simulink model "Just_The_Electrical_model"  (R2016a)
settings: Solver=VariableStepAuto  StartTime=0.0  StopTime=10.0  RelTol=1e-3
values from neighbouring files (symbols this model uses):
  BT = {}    [Electrical_model_settings.m]
  btc = {}    [Electrical_model_settings.m]
  col = {}    [Electrical_model_settings.m]
  elc = {}    [Electrical_model_settings.m]
  ess = {}    [Electrical_model_settings.m]
  fcc = {}    [Electrical_model_settings.m]
  flex = {}    [Electrical_model_settings.m]
  systemBase = {}    [Electrical_model_settings.m]
  wf = {}    [Electrical_model_settings.m]
  wt1 = {}    [Electrical_model_settings.m]
  wt2 = wt1    [Electrical_model_settings.m]
  wt3 = wt1    [Electrical_model_settings.m]
undefined symbols (not defined in the file or in its folder): avr, D1, Delta, DiscIntNeverNeededParam, f2ctrl, governor, interface, Lf1, sm, Ts, Ts_phy, Ts_sim, u0
libraries: powerlib x69, pwrsysBasic x68, simulink_extras x37, pwrsysVICtrl x22, powerlib_meascontrol x19, simulink x8, pwrsysVSrc x5, pwrsysTransf x5, pwrsys-matlab x1
(part 2 of 4)

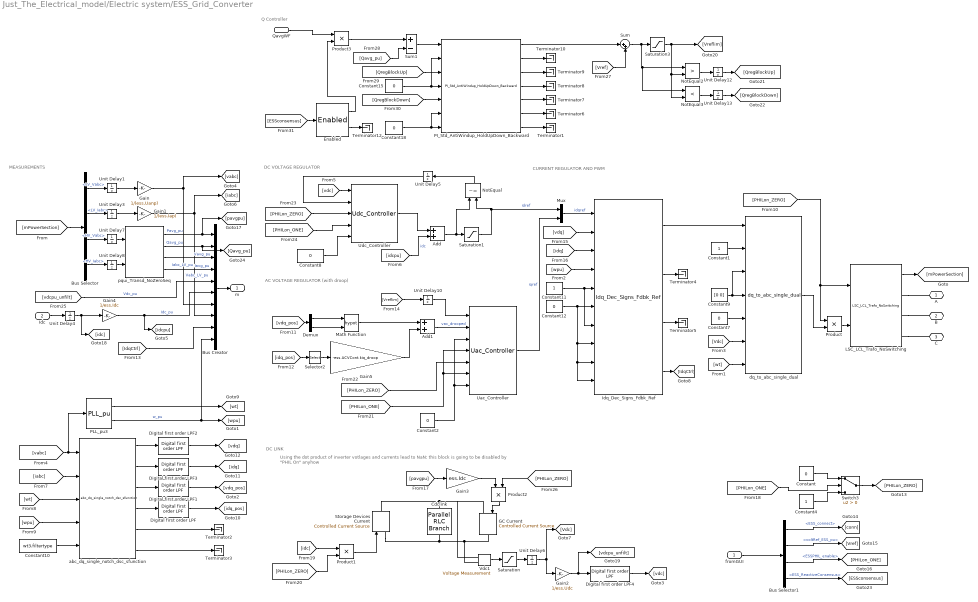
== system Just_The_Electrical_model/Electric system/ESS_Grid_Converter ==
  note: DC LINK
  note: Using the dot product of inverter votlages and currents lead to NaN: this block is going to be disabled by "PHIL On" anyhow
  note: MEASUREMENTS
  note: AC VOLTAGE REGULATOR (with droop)
  note: DC VOLTAGE REGULATOR
  note: CURRENT REGULATOR AND PWM
  note: Q Controller
  fromGUI : Inport
  Idc : Inport  Port=2
  QavgWF : Inport  Port=3
  Add : Sum
  Add1 : Sum
  Bus Creator : BusCreator  Inputs=10
  Bus Selector : BusSelector  OutputSignals=LV_Vabc,LV_Iabc,HV_Vabc,HV_Iabc
  Bus Selector1 : BusSelector  OutputSignals=ESS_connect,voltRef_ESS_pu,ESSPHIL_enable,ESS_ReactiveConsensus
  Cdclink : powerlib/Elements/Parallel RLC Branch  LConnTagsString=a  RConnTagsString=__new0  BranchType=RC  Resistance=1e6  Inductance=0  SetiL0=off  InitialCurrent=0  Capacitance=ess.Cdc  Setx0=on  InitialVoltage=ess.Udc  Measurements=None
  Constant{,2,15,18} (4 alike) : Constant  Value=0
  Constant1 : Constant  SampleTime=ess.Ts_control
  Constant10 : Constant  Value=wt3.filtertype  SampleTime=wt3.Ts_control
  Constant11 : Constant  SampleTime=ess.Ts_control
  Constant12 : Constant  Value=0  SampleTime=ess.Ts_control
  Constant4 : Constant
  Constant7 : Constant  Value=0  SampleTime=ess.Ts_control
  Constant8 : Constant  Value=0  SampleTime=ess.Ts_control
  Constant9 : Constant  Value=[0 0]  SampleTime=ess.Ts_control
  Demux : Demux  Outputs=2
  Digital first order LPF{,1..4} (5 alike) : pwrsysBasic/Digital first order LPF  Ts=ess.Ts_control  fcutout=ess.CurrCont.f_LPF_noise
  Enabled : pwrsysBasic/Enabled
  GC Current : powerlib/Electrical Sources/Controlled Current Source  Initialize=on  Source_Type=DC  Amplitude=0  Phase=0  Frequency=0  Measurements=None
  Gain : Gain  Gain=1/(ess.Uanp)
  Gain1 : Gain  Gain=1/(ess.Iap)
  Gain2 : Gain  Gain=1/ess.Udc
  Gain3 : Gain  Gain=ess.Idc
  Gain4 : Gain  Gain=1/ess.Idc
  Gain5 : Gain  Gain=-ess.ACVCont.kiq_droop
  Idq_Dec_Signs_Fdbk_Ref : pwrsysVICtrl/Idq_Dec_Signs_Fdbk_Ref  Ts=ess.Ts_control  fn=systemBase.fn  Kp=ess.CurrContSingle.kp  Ti=ess.CurrContSingle.Ti  L=ess.CurrCont.x  PI_max=ess.CurrCont.PImax  PI_min=ess.CurrCont.PImin  TrafoPhaseComp=0
  LSC_LCL_Trafo_NoSwitching : pwrsysVSrc/LSC_LCL_Trafo_NoSwitching  Sn=ess.Sn  fn=systemBase.fn  Uhv_ab=systemBase.Vn  Uab=ess.Un  lf2=ess.LCL.l2  rf2=ess.LCL.r2  Lf1=ess.LCL.L1  Rf1=ess.LCL.R1  Cf=ess.LCL.Cf  Rc=ess.LCL.Rf
  Math Function : Math  Operator=hypot  SaturateOnIntegerOverflow=on
  Mux : Mux  Inputs=2
  NotEqual : RelationalOperator  Operator=~=  OutDataTypeStr=boolean
  NotEqual2 : RelationalOperator  Operator=>  OutDataTypeStr=boolean
  NotEqual3 : RelationalOperator  Operator=<  OutDataTypeStr=boolean
  PI_Std_AntiWindup_HoldUpDown_Backward : pwrsysBasic/PI_Std_AntiWindup_HoldUpDown_Backward  Ts=ess.Ts_control  Kg=ess.Qctrl.Kg  Kp=ess.Qctrl.Kp  Ti=ess.Qctrl.Ti  outMax=ess.Qctrl.deltaUmaxPos  outMin=ess.Qctrl.deltaUmaxNeg
  PLL_pu3 : pwrsysBasic/PLL_pu  fn=systemBase.fn  Ts=ess.Ts_control  Kp_pll=90  Ki_pll=1200  Kd_pll=0  PLL_ini=60
  Product{,1..3} (4 alike) : Product
  Saturation : Saturate  UpperLimit=5*ess.Uanp  LowerLimit=0.25*ess.Uanp
  Saturation1 : Saturate  UpperLimit=ess.DCVCont.PImax  LowerLimit=ess.DCVCont.PImin
  Saturation3 : Saturate  UpperLimit=ess.Qctrl.Umax  LowerLimit=ess.Qctrl.Umin
  Selector2 : Selector  IndexMode=Zero-based  InputPortWidth=2  IndexOptions=Index vector (dialog)  Indices=1  OutputSizes=1
  Storage Devices Current : powerlib/Electrical Sources/Controlled Current Source  Initialize=on  Source_Type=DC  Amplitude=0  Phase=0  Frequency=0  Measurements=None
  Sum : Sum  Inputs=|++
  Sum1 : Sum  Inputs=+-
  Switch3 : Switch  Criteria=u2 > Threshold
  Terminator{1..10,12} (11 alike) : Terminator
  Uac_Controller : pwrsysVICtrl/Uac_Controller  Ts=ess.Ts_control  Kg=ess.ACVCont.kg  Kp=ess.ACVCont.kp  Ti=ess.ACVCont.Ti  PI_max=ess.ACVCont.PImax  PI_min=ess.ACVCont.PImin
  Udc_Controller : pwrsysVICtrl/Udc_Controller  Ts=ess.Ts_control  Kp=ess.DCVContSingle.kp  Ti=ess.DCVContSingle.Ti  PI_max=ess.DCVCont.PImax  PI_min=ess.DCVCont.PImin
  Unit Delay{1,3,7..8} (4 alike) : UnitDelay  InitialCondition=[0 0 0]  SampleTime=ess.Ts_control
  Unit Delay10 : UnitDelay  InitialCondition=1  SampleTime=ess.Ts_control
  Unit Delay{4..5,12..13} (4 alike) : UnitDelay  SampleTime=ess.Ts_control
  Unit Delay6 : UnitDelay  InitialCondition=1  SampleTime=ess.Ts_control
  Vdc1 : powerlib/Measurements/Voltage Measurement  PhasorSimulation=off  OutputType=Complex  PSBequivalent=0
  abc_dq_single_notch_dsc_sfunction : pwrsysTransf/abc_dq_single_notch_dsc_sfunction  Ts=ess.Ts_control  fn=2*systemBase.fn  zeta=ess.CurrCont.zeta
  dq_to_abc_single_dual : pwrsysVICtrl/dq_to_abc_single_dual  Ts=ess.Ts_control  Uabp=ess.Uabp
  pqui_Transd_NoZeroSeq : pwrsysBasic/pqui_Transd_NoZeroSeq  Sn=ess.Sn  Uanp=systemBase.Vn*(2/3)^0.5  Iap=ess.Iap*(ess.Un/systemBase.Vn)
  A : PMIOPort  Port=1  Side=Right
  B : PMIOPort  Port=2  Side=Right
  C : PMIOPort  Port=3  Side=Right
  m : Outport
  wires:
  Bus Selector/1 -> Unit Delay1/1  "<LV_Vabc>"
  [idq_pos] -> Selector2/1
  Gain1/1 -> Bus Creator/8, [iabc]  "Iabc_LV_pu"
  Bus Selector/2 -> Unit Delay3/1  "<LV_Iabc>"
  Gain5/1 -> Add1/2
  Math Function/1 -> Add1/1
  [PHILon_ONE] -> Uac_Controller/6, Uac_Controller/4
  Add1/1 -> Uac_Controller/2  "vac_drooped"
  [Vreflim] -> Unit Delay10/1
  [mPowerSection] -> Bus Selector/1
  Gain/1 -> Bus Creator/7, [vabc]  "Vabc_LV_pu"
  [PHILon_ZERO] -> Uac_Controller/5
  Constant8/1 -> Udc_Controller/5
  NotEqual/1 -> Unit Delay5/1
  [vdc] -> Udc_Controller/1
  Unit Delay5/1 -> Udc_Controller/2
  Saturation1/1 -> NotEqual/2, Mux/1  "idref"
  [idcpu] -> Add/2  "idc"
  Udc_Controller/1 -> Add/1
  Add/1 -> NotEqual/1, Saturation1/1
  [PHILon_ZERO] -> Udc_Controller/3
  [idq] -> Idq_Dec_Signs_Fdbk_Ref/3
  [Vdc] -> dq_to_abc_single_dual/6
  [wpu] -> Idq_Dec_Signs_Fdbk_Ref/4
  dq_to_abc_single_dual/1 -> Product/2
  Mux/1 -> Idq_Dec_Signs_Fdbk_Ref/1  "idqref"
  [wt] -> dq_to_abc_single_dual/7
  Constant10/1 -> abc_dq_single_notch_dsc_sfunction/5
  Bus Selector/3 -> Unit Delay7/1  "<HV_Vabc>"
  Bus Selector/4 -> Unit Delay8/1  "<HV_Iabc>"
  pqui_Transd_NoZeroSeq/1 -> [pavgpu], Bus Creator/1  "Pavg_pu"
  pqui_Transd_NoZeroSeq/2 -> [Qavg_pu], Bus Creator/2  "Qavg_pu"
  pqui_Transd_NoZeroSeq/3 -> Bus Creator/3  "Vavg_pu"
  pqui_Transd_NoZeroSeq/4 -> Bus Creator/4  "Iavg_pu"
  Bus Creator/1 -> m/1
  [vdcpu_unfilt] -> Bus Creator/5  "Vdc_pu"
  Gain4/1 -> [idcpu], Bus Creator/6  "Idc_pu"
  PLL_pu3/2 -> Bus Creator/10, [wpu]  "w_pu"
  PLL_pu3/1 -> [wt]
  Uac_Controller/1 -> Mux/2  "iqref"
  LSC_LCL_Trafo_NoSwitching/1 -> [mPowerSection]
  Unit Delay1/1 -> Gain/1
  Unit Delay3/1 -> Gain1/1
  Unit Delay8/1 -> pqui_Transd_NoZeroSeq/2
  Unit Delay7/1 -> pqui_Transd_NoZeroSeq/1
  Unit Delay10/1 -> Uac_Controller/1
  abc_dq_single_notch_dsc_sfunction/6 -> Terminator3/1
  abc_dq_single_notch_dsc_sfunction/5 -> Terminator2/1
  Selector2/1 -> Gain5/1
  Idq_Dec_Signs_Fdbk_Ref/2 -> Terminator4/1
  [vdq] -> Idq_Dec_Signs_Fdbk_Ref/2
  Constant1/1 -> dq_to_abc_single_dual/2
  Constant7/1 -> dq_to_abc_single_dual/5
  Constant9/1 -> dq_to_abc_single_dual/4, dq_to_abc_single_dual/3
  Constant11/1 -> Idq_Dec_Signs_Fdbk_Ref/7, Idq_Dec_Signs_Fdbk_Ref/5
  Constant12/1 -> Idq_Dec_Signs_Fdbk_Ref/8, Idq_Dec_Signs_Fdbk_Ref/9, Idq_Dec_Signs_Fdbk_Ref/10, Idq_Dec_Signs_Fdbk_Ref/6
  Idq_Dec_Signs_Fdbk_Ref/3 -> Terminator5/1
  Idq_Dec_Signs_Fdbk_Ref/4 -> [IdqCtrl]
  [IdqCtrl] -> Bus Creator/9
  Idq_Dec_Signs_Fdbk_Ref/1 -> dq_to_abc_single_dual/1
  [wt] -> abc_dq_single_notch_dsc_sfunction/3
  [wpu] -> abc_dq_single_notch_dsc_sfunction/4
  abc_dq_single_notch_dsc_sfunction/1 -> Digital first order LPF2/1
  [vabc] -> abc_dq_single_notch_dsc_sfunction/1, PLL_pu3/1
  [iabc] -> abc_dq_single_notch_dsc_sfunction/2
  abc_dq_single_notch_dsc_sfunction/3 -> Digital first order LPF1/1
  abc_dq_single_notch_dsc_sfunction/4 -> Digital first order LPF/1
  abc_dq_single_notch_dsc_sfunction/2 -> Digital first order LPF3/1
  Digital first order LPF/1 -> [idq_pos]
  Digital first order LPF1/1 -> [vdq_pos]
  [vdq_pos] -> Demux/1
  Demux/1 -> Math Function/1
  Demux/2 -> Math Function/2
  Digital first order LPF2/1 -> [vdq]
  Digital first order LPF3/1 -> [idq]
  fromGUI/1 -> Bus Selector1/1
  Bus Selector1/1 -> [conn]  "<ESS_connect>"
  Bus Selector1/2 -> [Vref]  "<voltRef_ESS_pu>"
  Idc/1 -> Unit Delay4/1
  Bus Selector1/3 -> [PHILon_ONE]  "<ESSPHIL_enable>"
  Unit Delay4/1 -> [idc], Gain4/1
  Constant/1 -> Switch3/1
  [PHILon_ONE] -> Switch3/2
  Constant4/1 -> Switch3/3
  Switch3/1 -> [PHILon_ZERO]
  [PHILon_ZERO] -> LSC_LCL_Trafo_NoSwitching/1, Product/1
  Product/1 -> LSC_LCL_Trafo_NoSwitching/2
  Gain3/1 -> Product2/1
  [pavgpu] -> Gain3/1
  [idc] -> Product1/1
  Product1/1 -> Storage Devices Current/1
  [PHILon_ZERO] -> Product1/2
  Constant2/1 -> Uac_Controller/3, Uac_Controller/7
  [PHILon_ONE] -> Udc_Controller/4
  Vdc1/1 -> Saturation/1
  Saturation/1 -> Unit Delay6/1
  Unit Delay6/1 -> [Vdc], Gain2/1
  Gain2/1 -> [vdcpu_unfilt], Digital first order LPF4/1
  Digital first order LPF4/1 -> [vdc]
  Product2/1 -> GC Current/1
  [PHILon_ZERO] -> Product2/2
  [Vref] -> Sum/2
  Sum/1 -> NotEqual3/1, NotEqual2/1, Saturation3/1
  Saturation3/1 -> NotEqual3/2, NotEqual2/2, [Vreflim]
  [Qavg_pu] -> Sum1/2
  [ESSconsensus] -> Enabled/1
  [QregBlockUp] -> PI_Std_AntiWindup_HoldUpDown_Backward/3
  Constant15/1 -> PI_Std_AntiWindup_HoldUpDown_Backward/2, PI_Std_AntiWindup_HoldUpDown_Backward/4
  [QregBlockDown] -> PI_Std_AntiWindup_HoldUpDown_Backward/5
  Constant18/1 -> PI_Std_AntiWindup_HoldUpDown_Backward/6, PI_Std_AntiWindup_HoldUpDown_Backward/7
  PI_Std_AntiWindup_HoldUpDown_Backward/7 -> Terminator1/1
  PI_Std_AntiWindup_HoldUpDown_Backward/6 -> Terminator6/1
  PI_Std_AntiWindup_HoldUpDown_Backward/5 -> Terminator7/1
  PI_Std_AntiWindup_HoldUpDown_Backward/4 -> Terminator8/1
  PI_Std_AntiWindup_HoldUpDown_Backward/3 -> Terminator9/1
  PI_Std_AntiWindup_HoldUpDown_Backward/2 -> Terminator10/1
  NotEqual2/1 -> Unit Delay12/1
  Unit Delay12/1 -> [QregBlockUp]
  NotEqual3/1 -> Unit Delay13/1
  Unit Delay13/1 -> [QregBlockDown]
  PI_Std_AntiWindup_HoldUpDown_Backward/1 -> Sum/1
  Bus Selector1/4 -> [ESSconsensus]  "<ESS_ReactiveConsensus>"
  Sum1/1 -> PI_Std_AntiWindup_HoldUpDown_Backward/1
  Enabled/2 -> Terminator12/1
  Product3/1 -> Sum1/1
  QavgWF/1 -> Product3/1
  Enabled/1 -> Product3/2
  connections:
  LSC_LCL_Trafo_NoSwitching/RConn3 -- C/RConn1
  LSC_LCL_Trafo_NoSwitching/RConn1 -- A/RConn1
  LSC_LCL_Trafo_NoSwitching/RConn2 -- B/RConn1
  Storage Devices Current/RConn1 -- Vdc1/LConn1 -- GC Current/LConn1 -- Cdclink/LConn1
  GC Current/RConn1 -- Vdc1/LConn2 -- Storage Devices Current/LConn1 -- Cdclink/RConn1

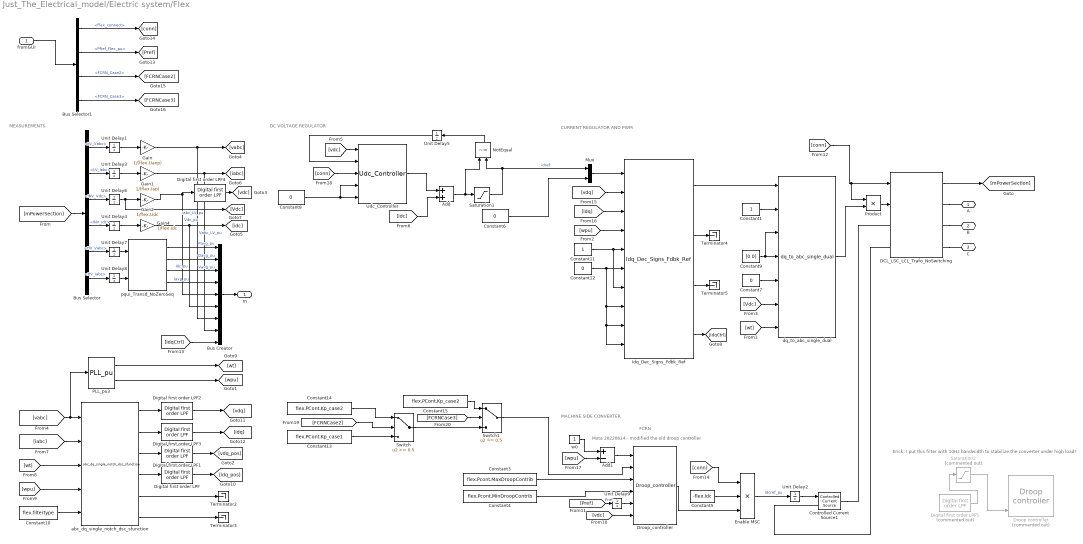
== system Just_The_Electrical_model/Electric system/Flex ==
  note: FCRN
  note: Mota 20220614 - modified the old droop controller
  note: Erick: I put this filter with 10Hz bandwidth to stabilize the converter under high load!
  note: MEASUREMENTS
  note: MACHINE SIDE CONVERTER
  note: DC VOLTAGE REGULATOR
  note: CURRENT REGULATOR AND PWM
  fromGUI : Inport
  Add : Sum
  Add1 : Sum  Inputs=+-
  Bus Creator : BusCreator  Inputs=9
  Bus Selector : BusSelector  OutputSignals=LV_Vabc,LV_Iabc,INV_Vdc,INV_Idc,HV_Vabc,HV_Iabc
  Bus Selector1 : BusSelector  OutputSignals=Flex_connect,PRef_Flex_pu,FCRN_Case2,FCRN_Case3
  Constant1 : Constant  SampleTime=flex.Ts_control
  Constant10 : Constant  Value=flex.filtertype  SampleTime=flex.Ts_control
  Constant11 : Constant  SampleTime=flex.Ts_control
  Constant{6..8,12} (4 alike) : Constant  Value=0  SampleTime=flex.Ts_control
  Constant13 : Constant  Value=flex.PCont.Kp_case1  SampleTime=-1
  Constant14 : Constant  Value=flex.PCont.Kp_case2  SampleTime=-1
  Constant15 : Constant  Value=flex.PCont.Kp_case2  SampleTime=-1
  Constant3 : Constant  Value=flex.Pcont.MaxDroopContrib  SampleTime=flex.Ts_control
  Constant4 : Constant  Value=flex.Pcont.MinDroopContrib  SampleTime=flex.Ts_control
  Constant5 : Constant  Value=-flex.Idc  SampleTime=flex.Ts_control
  Constant9 : Constant  Value=[0 0]  SampleTime=flex.Ts_control
  Controlled Current Source1 : powerlib/Electrical Sources/Controlled Current Source  Initialize=on  Source_Type=DC  Amplitude=0  Phase=0  Frequency=50  Measurements=None
  DCL_LSC_LCL_Trafo_NoSwitching : pwrsysVSrc/DCL_LSC_LCL_Trafo_NoSwitching  Sn=flex.Sn  fn=systemBase.fn  Uhv_ab=systemBase.Vn  Uab=flex.Un  lf2=flex.LCL.l2  rf2=flex.LCL.r2  Lf1=flex.LCL.L1  Rf1=flex.LCL.R1  Cf=flex.LCL.Cf  Rc=flex.LCL.Rf  Cdc=flex.Cdc  Udc0=flex.Udc  Tsm=flex.Ts_control  Tstart=flex.DCVCont.Start
  Digital first order LPF : pwrsysBasic/Digital first order LPF  Ts=wt1.Ts_control  fcutout=wt1.CurrCont.f_LPF_noise
  Digital first order LPF1 : pwrsysBasic/Digital first order LPF  Ts=flex.Ts_control  fcutout=flex.CurrCont.f_LPF_noise
  Digital first order LPF2 : pwrsysBasic/Digital first order LPF  Ts=flex.Ts_control  fcutout=flex.CurrCont.f_LPF_noise
  Digital first order LPF3 : pwrsysBasic/Digital first order LPF  Ts=wt1.Ts_control  fcutout=wt1.CurrCont.f_LPF_noise
  Digital first order LPF4 : pwrsysBasic/Digital first order LPF  Ts=flex.Ts_control  fcutout=flex.CurrCont.f_LPF_noise
  Digital first order LPF5 : pwrsysBasic/Digital first order LPF  Commented=on  Ts=flex.Ts_control  fcutout=10
  Droop controller : pwrsysBasic/Droop controller  Commented=on  Refmax=1  Refmin=0  Ts=flex.Ts_control  Kp=flex.PCont.Kp  Kd=flex.PCont.Kd  Tr=flex.PCont.Tr  flp=flex.PCont.flp  DB=flex.PCont.DB
  "Droop_controller " : pwrsysBasic/Droop_controller   Ts=flex.Ts_control  Outmax=flex.cosphi  Outmin=0  Refmax=flex.cosphi  Refmin=0  Kd=flex.PCont.Kd  Tr=flex.PCont.Tr  flp=flex.PCont.flp  DB=flex.PCont.DB  flp_comp=10  Compmax=1.2  Compini=1  Compmin=0.8
  Enable MSC : Product  Inputs=***
  Gain : Gain  Gain=1/(flex.Uanp)
  Gain1 : Gain  Gain=1/(flex.Iap)
  Gain2 : Gain  Gain=1/flex.Udc
  Gain4 : Gain  Gain=1/flex.Idc
  Idq_Dec_Signs_Fdbk_Ref : pwrsysVICtrl/Idq_Dec_Signs_Fdbk_Ref  Ts=flex.Ts_control  fn=systemBase.fn  Kp=flex.CurrContSingle.kp  Ti=flex.CurrContSingle.Ti  L=flex.CurrCont.x  PI_max=flex.CurrCont.PImax  PI_min=flex.CurrCont.PImin  TrafoPhaseComp=0
  Mux : Mux  Inputs=2
  NotEqual : RelationalOperator  Operator=~=  OutDataTypeStr=boolean
  PLL_pu3 : pwrsysBasic/PLL_pu  fn=systemBase.fn  Ts=flex.Ts_control  Kp_pll=90  Ki_pll=1200  Kd_pll=0  PLL_ini=60
  Product : Product
  Saturation1 : Saturate  UpperLimit=flex.DCVCont.PImax  LowerLimit=flex.DCVCont.PImin
  Saturation2 : Saturate  Commented=on  UpperLimit=1.2  LowerLimit=0.8
  Switch : Switch  Threshold=0.5
  Switch1 : Switch  Threshold=0.5
  Terminator{2..5} (4 alike) : Terminator
  Udc_Controller : pwrsysVICtrl/Udc_Controller  Ts=flex.Ts_control  Kp=flex.DCVContDual.kp  Ti=flex.DCVContDual.Ti  PI_max=flex.DCVCont.PImax  PI_min=flex.DCVCont.PImin
  Unit Delay{1,3,7..8} (4 alike) : UnitDelay  InitialCondition=[0 0 0]  SampleTime=flex.Ts_control
  Unit Delay{2,4..5,9} (4 alike) : UnitDelay  SampleTime=flex.Ts_control
  Unit Delay6 : UnitDelay  InitialCondition=1  SampleTime=flex.Ts_control
  abc_dq_single_notch_dsc_sfunction : pwrsysTransf/abc_dq_single_notch_dsc_sfunction  Ts=flex.Ts_control  fn=2*systemBase.fn  zeta=flex.CurrCont.zeta
  dq_to_abc_single_dual : pwrsysVICtrl/dq_to_abc_single_dual  Ts=flex.Ts_control  Uabp=flex.Uabp
  pqui_Transd_NoZeroSeq : pwrsysBasic/pqui_Transd_NoZeroSeq  Sn=flex.Sn  Uanp=systemBase.Vn*(2/3)^0.5  Iap=flex.Iap*(flex.Un/systemBase.Vn)
  w0 : Constant  SampleTime=flex.Ts_control
  A : PMIOPort  Port=1  Side=Right
  B : PMIOPort  Port=2  Side=Right
  C : PMIOPort  Port=3  Side=Right
  m : Outport
  wires:
  Bus Selector/1 -> Unit Delay1/1  "<LV_Vabc>"
  Unit Delay2/1 -> Controlled Current Source1/1
  Gain1/1 -> Bus Creator/8, [iabc]  "Iabc_LV_pu"
  Bus Selector/2 -> Unit Delay3/1  "<LV_Iabc>"
  Constant6/1 -> Mux/2
  Constant5/1 -> Enable MSC/2
  [mPowerSection] -> Bus Selector/1
  Enable MSC/1 -> Unit Delay2/1  "Idcref_pu"
  Gain/1 -> Bus Creator/7, [vabc]  "Vabc_LV_pu"
  Constant8/1 -> Udc_Controller/4, Udc_Controller/5
  NotEqual/1 -> Unit Delay5/1
  [vdc] -> Udc_Controller/1
  Unit Delay5/1 -> Udc_Controller/2
  Saturation1/1 -> NotEqual/2, Mux/1  "idref"
  [idc] -> Add/2
  Udc_Controller/1 -> Add/1
  Add/1 -> NotEqual/1, Saturation1/1
  [conn] -> Udc_Controller/3
  [idq] -> Idq_Dec_Signs_Fdbk_Ref/3
  [Vdc] -> dq_to_abc_single_dual/6
  [wpu] -> Idq_Dec_Signs_Fdbk_Ref/4
  dq_to_abc_single_dual/1 -> Product/2
  Mux/1 -> Idq_Dec_Signs_Fdbk_Ref/1
  [conn] -> Product/1, DCL_LSC_LCL_Trafo_NoSwitching/1
  [Pref] -> Unit Delay9/1  "Pref"
  [wt] -> dq_to_abc_single_dual/7
  Constant10/1 -> abc_dq_single_notch_dsc_sfunction/5
  Bus Selector/5 -> Unit Delay7/1  "<HV_Vabc>"
  Bus Selector/6 -> Unit Delay8/1  "<HV_Iabc>"
  pqui_Transd_NoZeroSeq/1 -> Bus Creator/1  "Pavg_pu"
  pqui_Transd_NoZeroSeq/2 -> Bus Creator/2  "Qavg_pu"
  pqui_Transd_NoZeroSeq/3 -> Bus Creator/3  "Vavg_pu"
  pqui_Transd_NoZeroSeq/4 -> Bus Creator/4  "Iavg_pu"
  Bus Creator/1 -> m/1
  Bus Selector/3 -> Unit Delay6/1  "<INV_Vdc>"
  Gain2/1 -> Bus Creator/5, Digital first order LPF4/1  "Vdc_pu"
  Gain4/1 -> [idc], Bus Creator/6  "Idc_pu"
  Bus Selector/4 -> Unit Delay4/1  "<INV_Idc>"
  PLL_pu3/2 -> [wpu]
  PLL_pu3/1 -> [wt]
  DCL_LSC_LCL_Trafo_NoSwitching/1 -> [mPowerSection]
  Unit Delay1/1 -> Gain/1
  Unit Delay3/1 -> Gain1/1
  Unit Delay4/1 -> Gain4/1
  Unit Delay8/1 -> pqui_Transd_NoZeroSeq/2
  Unit Delay6/1 -> [Vdc], Gain2/1
  Unit Delay7/1 -> pqui_Transd_NoZeroSeq/1
  Unit Delay9/1 -> "Droop_controller "/5
  abc_dq_single_notch_dsc_sfunction/6 -> Terminator3/1
  abc_dq_single_notch_dsc_sfunction/5 -> Terminator2/1
  Idq_Dec_Signs_Fdbk_Ref/2 -> Terminator4/1
  [vdq] -> Idq_Dec_Signs_Fdbk_Ref/2
  Constant1/1 -> dq_to_abc_single_dual/2
  Constant7/1 -> dq_to_abc_single_dual/5
  Constant9/1 -> dq_to_abc_single_dual/4, dq_to_abc_single_dual/3
  Constant11/1 -> Idq_Dec_Signs_Fdbk_Ref/7, Idq_Dec_Signs_Fdbk_Ref/5
  Constant12/1 -> Idq_Dec_Signs_Fdbk_Ref/8, Idq_Dec_Signs_Fdbk_Ref/9, Idq_Dec_Signs_Fdbk_Ref/10, Idq_Dec_Signs_Fdbk_Ref/6
  Idq_Dec_Signs_Fdbk_Ref/3 -> Terminator5/1
  Idq_Dec_Signs_Fdbk_Ref/4 -> [IdqCtrl]
  [IdqCtrl] -> Bus Creator/9
  Idq_Dec_Signs_Fdbk_Ref/1 -> dq_to_abc_single_dual/1
  [wt] -> abc_dq_single_notch_dsc_sfunction/3
  [wpu] -> abc_dq_single_notch_dsc_sfunction/4
  abc_dq_single_notch_dsc_sfunction/1 -> Digital first order LPF2/1
  [vabc] -> abc_dq_single_notch_dsc_sfunction/1, PLL_pu3/1
  [iabc] -> abc_dq_single_notch_dsc_sfunction/2
  abc_dq_single_notch_dsc_sfunction/3 -> Digital first order LPF1/1
  abc_dq_single_notch_dsc_sfunction/4 -> Digital first order LPF/1
  abc_dq_single_notch_dsc_sfunction/2 -> Digital first order LPF3/1
  Digital first order LPF/1 -> [idq_pos]
  Digital first order LPF1/1 -> [vdq_pos]
  Digital first order LPF2/1 -> [vdq]
  Digital first order LPF3/1 -> [idq]
  Digital first order LPF4/1 -> [vdc]
  Saturation2/1 -> Droop controller/3
  Digital first order LPF5/1 -> Saturation2/1
  fromGUI/1 -> Bus Selector1/1
  Bus Selector1/2 -> [Pref]  "<PRef_Flex_pu>"
  Bus Selector1/1 -> [conn]  "<Flex_connect>"
  [conn] -> Enable MSC/1
  [wpu] -> Add1/2
  w0/1 -> Add1/1
  Product/1 -> DCL_LSC_LCL_Trafo_NoSwitching/2
  Switch1/1 -> "Droop_controller "/2
  Constant3/1 -> "Droop_controller "/3
  Constant4/1 -> "Droop_controller "/4
  Add1/1 -> "Droop_controller "/1
  [vdc] -> "Droop_controller "/6
  "Droop_controller "/1 -> Enable MSC/3
  Bus Selector1/3 -> [FCRNCase2]  "<FCRN_Case2>"
  Bus Selector1/4 -> [FCRNCase3]  "<FCRN_Case3>"
  [FCRNCase2] -> Switch/2
  Constant13/1 -> Switch/3
  Constant14/1 -> Switch/1
  Switch/1 -> Switch1/3
  [FCRNCase3] -> Switch1/2
  Constant15/1 -> Switch1/1
  connections:
  Controlled Current Source1/RConn1 -- DCL_LSC_LCL_Trafo_NoSwitching/LConn1
  DCL_LSC_LCL_Trafo_NoSwitching/RConn3 -- C/RConn1
  DCL_LSC_LCL_Trafo_NoSwitching/RConn1 -- A/RConn1
  DCL_LSC_LCL_Trafo_NoSwitching/RConn2 -- B/RConn1
  Controlled Current Source1/LConn1 -- DCL_LSC_LCL_Trafo_NoSwitching/LConn2

== system Just_The_Electrical_model/Electric system/Power Management System ==
  note: Datalog
  w : Inport
  fromDCgrid : Inport  Port=2
  resetInt : Inport  Port=3
  Bus Creator : BusCreator  Inputs=5
  Bus Selector1 : BusSelector  OutputSignals=FC_Pdc_pu,EL_Pdc_pu
  Constant : Constant  Value=0.025
  Constant1 : Constant  SampleTime=-1
  Constant2 : Constant  Value=-0.025
  Data Type Conversion1 : DataTypeConversion  OutDataTypeStr=double  RndMeth=Round
  Data Type Conversion6 : DataTypeConversion  OutDataTypeStr=double  RndMeth=Round
  Digital first order LPF1 : pwrsysBasic/Digital first order LPF  Ts=Ts  fcutout=0.3181
  Digital first order LPF8 : pwrsysBasic/Digital first order LPF  Ts=Ts  fcutout=0.3181
  Discrete-Time Integrator : DiscreteIntegrator  ExternalReset=rising  InitialConditionSetting=State (most efficient)  SampleTime=Ts  LimitOutput=on  UpperSaturationLimit=f2ctrl.PImax  LowerSaturationLimit=f2ctrl.PImin  ICPrevOutput=DiscIntNeverNeededParam  ICPrevScaledInput=DiscIntNeverNeededParam
  Gain : Gain  Gain=systemBase.Pn
  Gain1 : Gain  Gain=1/fcc.Pn
  Gain2 : Gain  Gain=1/elc.Pn
  Gain3 : Gain  Gain=fcc.Pn
  Gain4 : Gain  Gain=elc.Pn
  Gain5 : Gain  Gain=1/sm.Sn
  Interval Test : simulink/Logic and Bit Operations/Interval Test  IntervalClosedRight=on  uplimit=0.1e6  IntervalClosedLeft=on  lowlimit=-0.1e6  OutDataTypeStr=boolean
  Interval Test2 : simulink/Logic and Bit Operations/Interval Test  IntervalClosedRight=on  uplimit=btc.Pfdroop.DB*0.8  IntervalClosedLeft=on  lowlimit=-btc.Pfdroop.DB*0.8  OutDataTypeStr=boolean
  Ki : Gain  Gain=f2ctrl.Ki
  Kp : Gain  Gain=f2ctrl.Kp
  Logical Operator : Logic  Operator=NOT  AllPortsSameDT=off  OutDataTypeStr=boolean
  Logical Operator1 : Logic  Operator=NOT  AllPortsSameDT=off  OutDataTypeStr=boolean
  Off Delay : powerlib_meascontrol/Logic/On Delay  DelayType=On delay  delay=f2ctrl.offdelay  ic=0  Ts=Ts
  On Delay : powerlib_meascontrol/Logic/On Delay  DelayType=On delay  delay=f2ctrl.ondelay  ic=0  Ts=Ts
  P ES2 error : Sum  Inputs=--+
  Product{1..5} (5 alike) : Product
  Psec_unlim : Sum
  Relational Operator : RelationalOperator  Operator===  OutDataTypeStr=boolean
  Relational Operator1 : RelationalOperator  Operator=>  OutDataTypeStr=boolean
  Relational Operator2 : RelationalOperator  Operator=<  OutDataTypeStr=boolean
  S-R Flip-Flop : simulink_extras/Flip Flops/S-R Flip-Flop  initial_condition=0
  Saturation : Saturate  UpperLimit=1  LowerLimit=0
  Saturation1 : Saturate  UpperLimit=0  LowerLimit=-1
  Saturation2 : Saturate  UpperLimit=f2ctrl.PImax  LowerLimit=f2ctrl.PImin
  Terminator : Terminator
  Unit Delay2 : UnitDelay  InitialCondition=1  SampleTime=-1
  f error : Sum  Inputs=+-
  guiPushButtonInterface : Subsystem
  m : Outport
  wires:
  Constant1/1 -> f error/1
  Product3/1 -> Gain5/1  "Psec_SIgt"
  P ES2 error/1 -> Interval Test/1, Product3/2  "Pes2error"
  Saturation2/1 -> [Psec_pusysb], Relational Operator/1, Gain/1  "Psec_pu"
  Interval Test2/1 -> Logical Operator1/1, Off Delay/1
  Off Delay/1 -> S-R Flip-Flop/2
  Logical Operator1/1 -> On Delay/1
  f error/1 -> Product2/2, Interval Test2/1  "werr"
  Interval Test/1 -> Logical Operator/1
  Logical Operator/1 -> Product3/1
  On Delay/1 -> S-R Flip-Flop/1
  Bus Creator/1 -> m/1  "Sec"
  [Psec_ely] -> Bus Creator/3  "Psec_ely"
  [Psec_fc] -> Bus Creator/4  "Psec_fc"
  [Psec_pusysb] -> Bus Creator/1  "Psec_pusysb"
  [Psec_gt] -> Bus Creator/2  "Psec_gt"
  [Sec_active] -> Bus Creator/5  "Sec_active"
  Gain1/1 -> Saturation/1
  Gain/1 -> Gain2/1, Gain1/1, P ES2 error/3  "Psec_SI"
  Gain2/1 -> Saturation1/1
  Gain4/1 -> P ES2 error/2  "Pfc_SI"
  Gain5/1 -> [Psec_gt]
  w/1 -> f error/2
  S-R Flip-Flop/1 -> Data Type Conversion6/1
  Ki/1 -> Product1/2
  Kp/1 -> Psec_unlim/2
  Discrete-Time Integrator/1 -> Psec_unlim/1
  Psec_unlim/1 -> Saturation2/1, Relational Operator/2
  Relational Operator/1 -> Unit Delay2/1
  Unit Delay2/1 -> Data Type Conversion1/1
  Product2/1 -> Kp/1, Ki/1
  Product1/1 -> Discrete-Time Integrator/1
  S-R Flip-Flop/2 -> Terminator/1
  Data Type Conversion6/1 -> [Sec_active], Product2/1
  Data Type Conversion1/1 -> Product1/1
  fromDCgrid/1 -> Bus Selector1/1
  Bus Selector1/1 -> Digital first order LPF8/1  "<FC_Pdc_pu>"
  Bus Selector1/2 -> Digital first order LPF1/1  "<EL_Pdc_pu>"
  Gain3/1 -> P ES2 error/1  "Pely_SI"
  resetInt/1 -> guiPushButtonInterface/1(In1)
  Digital first order LPF8/1 -> Gain3/1
  Digital first order LPF1/1 -> Gain4/1
  guiPushButtonInterface/1(Out1) -> Discrete-Time Integrator/2
  Saturation/1 -> Relational Operator1/1, Product4/2
  Saturation1/1 -> Relational Operator2/1, Product5/1
  Constant/1 -> Relational Operator1/2
  Relational Operator1/1 -> Product4/1
  Product4/1 -> [Psec_fc]
  Constant2/1 -> Relational Operator2/2
  Relational Operator2/1 -> Product5/2
  Product5/1 -> [Psec_ely]

== system Just_The_Electrical_model/Electric system/Reactive power sharing ==
  From GUI : Inport
  From WF : Inport  Port=2
  From GT : Inport  Port=3
  From ESS : Inport  Port=4
  From HIL : Inport  Port=5
  Bus Selector1 : BusSelector  OutputSignals=Qgen_pu
  Bus Selector13 : BusSelector  OutputSignals=WT1_connect,WT2_connect,WT3_connect,WF_ReactiveConsensus,GT_ReactiveConsensus,ESS_ReactiveConsensus,ESS_connect,ESSPHIL_enable
  Bus Selector2 : BusSelector  OutputSignals=Qavg_pu
  Bus Selector3 : BusSelector  OutputSignals=WT1.Qavg_pu
  Bus Selector4 : BusSelector  OutputSignals=WT2.Qavg_pu
  Bus Selector5 : BusSelector  OutputSignals=WT3.Qavg_pu
  Bus Selector6 : BusSelector  OutputSignals=Interface_Q_pu
  Digital first order LPF6 : pwrsysBasic/Digital first order LPF  Ts=Ts  fcutout=Qconsensus.QavgvCalcCutOutFreq
  Divide1 : Product  Inputs=*/
  Enabled : pwrsysBasic/Enabled
  Product{1..7,9..10,12} (10 alike) : Product
  Product8 : Product  Inputs=3
  Saturation1 : Saturate  UpperLimit=inf  LowerLimit=1
  Sum2 : Sum  Inputs=++++++
  Sum3 : Sum  Inputs=++++++
  QavgConsensus : Outport
  wires:
  From GUI/1 -> Bus Selector13/1
  Bus Selector13/1 -> [WT1connect]  "<WT1_connect>"
  Bus Selector13/2 -> [WT2connect]  "<WT2_connect>"
  Bus Selector13/3 -> [WT3connect]  "<WT3_connect>"
  Bus Selector3/1 -> Product1/2  "<Qavg_pu>"
  [WT1connect] -> Product4/1
  [WFconsensus] -> Product4/2
  Bus Selector4/1 -> Product5/2  "<Qavg_pu>"
  [WT2connect] -> Product6/1
  [WFconsensus] -> Product6/2
  From WF/1 -> Bus Selector5/1, Bus Selector4/1, Bus Selector3/1
  Bus Selector5/1 -> Product7/2  "<Qavg_pu>"
  [WT3connect] -> Product2/1
  [WFconsensus] -> Product2/2
  Product6/1 -> Sum2/5, Product5/1
  Product4/1 -> Sum2/4, Product1/1
  Digital first order LPF6/1 -> QavgConsensus/1
  Bus Selector13/4 -> [WFconsensus]  "<WF_ReactiveConsensus>"
  Bus Selector13/5 -> [GTconsensus]  "<GT_ReactiveConsensus>"
  From GT/1 -> Bus Selector1/1
  Bus Selector1/1 -> Product3/2  "<Qgen_pu>"
  [GTconsensus] -> Sum2/1, Product3/1
  From ESS/1 -> Bus Selector2/1
  Bus Selector13/7 -> [ESSconnect]  "<ESS_connect>"
  Bus Selector13/8 -> Enabled/1  "<ESSPHIL_enable>"
  [ESSconnect] -> Product8/1
  Enabled/1 -> [ESSPHIL_Enabled]
  Enabled/2 -> [ESSPHIL_Disabled]
  [ESSPHIL_Disabled] -> Product8/2
  Product8/1 -> Product9/1, Sum2/2
  Sum2/1 -> Saturation1/1
  Product3/1 -> Sum3/1
  Bus Selector2/1 -> Product9/2  "<Qavg_pu>"
  Product9/1 -> Sum3/2
  From HIL/1 -> Bus Selector6/1
  Bus Selector6/1 -> Product10/2  "<Interface_Q_pu>"
  Product10/1 -> Sum3/3
  Saturation1/1 -> Divide1/2
  Sum3/1 -> Divide1/1
  Divide1/1 -> Digital first order LPF6/1
  Bus Selector13/6 -> [ESSconsensus]  "<ESS_ReactiveConsensus>"
  [ESSconsensus] -> Product8/3
  [ESSPHIL_Enabled] -> Product12/1
  [ESSconsensus] -> Product12/2
  Product12/1 -> Product10/1, Sum2/3
  Product1/1 -> Sum3/4
  Product5/1 -> Sum3/5
  Product2/1 -> Sum2/6, Product7/1
  Product7/1 -> Sum3/6

== system Just_The_Electrical_model/Electric system/Rotation1 ==
  generator power (pu) : Inport
  driving torque (pu) : Inport  Port=2
  InitialSpeed : Inport  Port=3
  resetSpeed : Inport  Port=4
  Constant : Constant
  Constant1 : Constant  Value=-1
  Damping : Gain  Gain=sm.mechanicalDamping
  Discrete-Time Integrator : DiscreteIntegrator  IntegratorMethod=Integration: Trapezoidal  ExternalReset=rising  InitialConditionSource=external  SampleTime=Ts  LimitOutput=on  UpperSaturationLimit=sm.speedBlockingLimit  LowerSaturationLimit=-sm.speedBlockingLimit  ICPrevOutput=DiscIntNeverNeededParam  ICPrevScaledInput=DiscIntNeverNeededParam
  Divide : Product  Inputs=**
  Divide1 : Product  Inputs=*/
  Divide2 : Product  Inputs=*/
  Inertia : Constant  Value=sm.inertiaSeconds
  Memory : Memory
  Memory1 : Memory
  Saturation : Saturate  UpperLimit=inf  LowerLimit=sm.minSpeedForTorqueCalc
  Sum : Sum  Inputs=-+
  Sum3 : Sum  Inputs=-+
  Switch : Switch
  guiPushButtonInterface : Subsystem
  turbine speed (pu) : Outport
  mechanical torque (pu) : Outport  Port=2
  electric torque (pu) : Outport  Port=3
  wires:
  resetSpeed/1 -> guiPushButtonInterface/1(In1)
  Constant1/1 -> Switch/3
  Constant/1 -> Switch/1
  Switch/1 -> Divide/2
  Saturation/1 -> Divide/1
  Divide/1 -> Divide2/2
  InitialSpeed/1 -> Discrete-Time Integrator/3
  Discrete-Time Integrator/1 -> Memory/1, turbine speed (pu)/1, Damping/1  "w (pu)"
  Divide1/1 -> Discrete-Time Integrator/1
  Damping/1 -> Memory1/1  "damping torque (pu)"
  Inertia/1 -> Divide1/2
  Sum3/1 -> Divide1/1
  Divide2/1 -> Sum3/1, electric torque (pu)/1
  Sum/1 -> mechanical torque (pu)/1, Sum3/2  "accelarting torque"
  driving torque (pu)/1 -> Sum/2
  generator power (pu)/1 -> Divide2/1
  Memory/1 -> Saturation/1, Switch/2
  Memory1/1 -> Sum/1
  guiPushButtonInterface/1(Out1) -> Discrete-Time Integrator/2

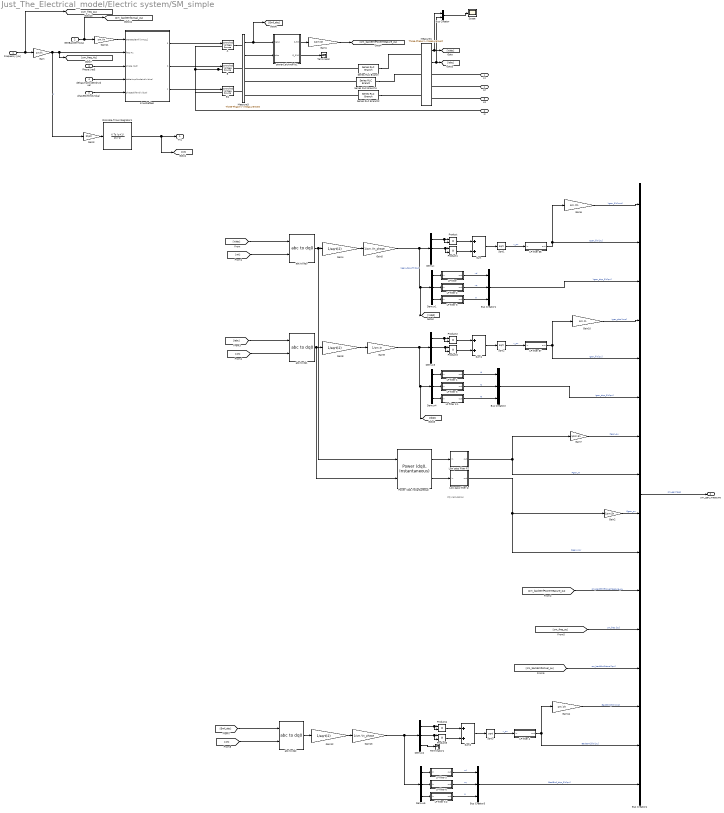
== system Just_The_Electrical_model/Electric system/SM_simple ==
  note: PQ calculation
  Frequency [pu] : Inport
  GenBackEmf [pu] : Inport  Port=2
  Phase [rad] : Inport  Port=3
  deltaAmplitudeIndividual : Inport  Port=4
  phaseSkiftIndividual : Inport  Port=5
  A : powerlib/Electrical Sources/Controlled Voltage Source  Initialize=off  Source_Type=DC  Amplitude=0  Phase=0  Frequency=0  Measurements=Voltage
  B : powerlib/Electrical Sources/Controlled Voltage Source  Initialize=off  Source_Type=DC  Amplitude=0  Phase=0  Frequency=0  Measurements=None
  B1 : powerlib/Electrical Sources/Controlled Voltage Source  Initialize=off  Source_Type=DC  Amplitude=0  Phase=0  Frequency=0  Measurements=Voltage
  Bus Creator : BusCreator  Inputs=2
  Bus Creator1 : BusCreator  Inputs=3
  Bus Creator2 : BusCreator  Inputs=3
  Bus Creator3 : BusCreator  Inputs=3
  Bus Creator4 : BusCreator  Inputs=16
  Demux{,1..5} (6 alike) : Demux  Outputs=3
  Discrete-Time Integrator1 : DiscreteIntegrator  IntegratorMethod=Integration: Trapezoidal  SampleTime=Ts  UpperSaturationLimit=sm.speedBlockingLimit  LowerSaturationLimit=-sm.speedBlockingLimit  ICPrevOutput=DiscIntNeverNeededParam  ICPrevScaledInput=DiscIntNeverNeededParam
  Gain : Gain  Gain=sm.fn
  Gain1 : Gain  Gain=1/sm.Sn
  Gain10 : Gain  Gain=sm.In
  Gain11 : Gain  Gain=sm.Vn
  Gain12 : Gain  Gain=1/sqrt(2)
  Gain13 : Gain  Gain=1/sm.Vn_phase
  Gain14 : Gain  Gain=sm.Vn
  Gain2 : Gain  Gain=1/sm.Sn
  Gain3 : Gain  Gain=2*pi()
  Gain4 : Gain  Gain=1/sqrt(2)
  Gain5 : Gain  Gain=1/sm.Vn_phase
  Gain6 : Gain  Gain=sm.Vn
  Gain7 : Gain  Gain=1/sm.Sn
  Gain8 : Gain  Gain=1/sqrt(2)
  Gain9 : Gain  Gain=1/sm.In
  "LP filter " : Subsystem  mask(Discrete first order low pass filter){tau=sm.V_measure_T, Ts=Ts, x0=avr.init, y0=avr.init}
      mask prompts: tau "Filter time constant [s]"; Ts "Sampling time [s]"; x0 "Initial input"; y0 "Initial output"
      mask help: Discrete first order low pass filter derived from a continous filter by bilinear transformation.
  LP filter 1 : Subsystem  mask(Discrete first order low pass filter){tau=sm.I_measure_T, Ts=Ts, x0=0, y0=0}
      mask prompts: tau "Filter time constant [s]"; Ts "Sampling time [s]"; x0 "Initial input"; y0 "Initial output"
      mask help: Discrete first order low pass filter derived from a continous filter by bilinear transformation.
  LP filter 2 : Subsystem  mask(Discrete first order low pass filter){tau=sm.V_measure_T, Ts=Ts, x0=avr.init, y0=avr.init}
      mask prompts: tau "Filter time constant [s]"; Ts "Sampling time [s]"; x0 "Initial input"; y0 "Initial output"
      mask help: Discrete first order low pass filter derived from a continous filter by bilinear transformation.
  LP filter 3 : Subsystem  mask(Discrete first order low pass filter){tau=sm.I_measure_T, Ts=Ts, x0=avr.init, y0=avr.init}
      mask prompts: tau "Filter time constant [s]"; Ts "Sampling time [s]"; x0 "Initial input"; y0 "Initial output"
      mask help: Discrete first order low pass filter derived from a continous filter by bilinear transformation.
  "LP filter 3 " : Subsystem  mask(Discrete first order low pass filter){tau=sm.V_measure_T, Ts=Ts, x0=avr.init, y0=avr.init}
      mask prompts: tau "Filter time constant [s]"; Ts "Sampling time [s]"; x0 "Initial input"; y0 "Initial output"
      mask help: Discrete first order low pass filter derived from a continous filter by bilinear transformation.
  LP filter 3 1 : Subsystem  mask(Discrete first order low pass filter){tau=sm.I_measure_T, Ts=Ts, x0=avr.init, y0=avr.init}
      mask prompts: tau "Filter time constant [s]"; Ts "Sampling time [s]"; x0 "Initial input"; y0 "Initial output"
      mask help: Discrete first order low pass filter derived from a continous filter by bilinear transformation.
  LP filter 3 2 : Subsystem  mask(Discrete first order low pass filter){tau=sm.V_measure_T, Ts=Ts, x0=avr.init, y0=avr.init}
      mask prompts: tau "Filter time constant [s]"; Ts "Sampling time [s]"; x0 "Initial input"; y0 "Initial output"
      mask help: Discrete first order low pass filter derived from a continous filter by bilinear transformation.
  LP filter 4 : Subsystem  mask(Discrete first order low pass filter){tau=sm.V_measure_T, Ts=Ts, x0=avr.init, y0=avr.init}
      mask prompts: tau "Filter time constant [s]"; Ts "Sampling time [s]"; x0 "Initial input"; y0 "Initial output"
      mask help: Discrete first order low pass filter derived from a continous filter by bilinear transformation.
  LP filter 5 : Subsystem  mask(Discrete first order low pass filter){tau=sm.V_measure_T, Ts=Ts, x0=avr.init, y0=avr.init}
      mask prompts: tau "Filter time constant [s]"; Ts "Sampling time [s]"; x0 "Initial input"; y0 "Initial output"
      mask help: Discrete first order low pass filter derived from a continous filter by bilinear transformation.
  LP filter 6 : Subsystem  mask(Discrete first order low pass filter){tau=sm.V_measure_T, Ts=Ts, x0=avr.init, y0=avr.init}
      mask prompts: tau "Filter time constant [s]"; Ts "Sampling time [s]"; x0 "Initial input"; y0 "Initial output"
      mask help: Discrete first order low pass filter derived from a continous filter by bilinear transformation.
  LP filter 66 : Subsystem  mask(Discrete first order low pass filter){tau=sm.V_measure_T, Ts=Ts, x0=avr.init, y0=avr.init}
      mask prompts: tau "Filter time constant [s]"; Ts "Sampling time [s]"; x0 "Initial input"; y0 "Initial output"
      mask help: Discrete first order low pass filter derived from a continous filter by bilinear transformation.
  LP filter 67 : Subsystem  mask(Discrete first order low pass filter){tau=sm.I_measure_T, Ts=Ts, x0=avr.init, y0=avr.init}
      mask prompts: tau "Filter time constant [s]"; Ts "Sampling time [s]"; x0 "Initial input"; y0 "Initial output"
      mask help: Discrete first order low pass filter derived from a continous filter by bilinear transformation.
  Low pass filter P1 : Subsystem  mask(Discrete first order low pass filter){tau=sm.P_measure, Ts=Ts, x0=0, y0=0}
      mask prompts: tau "Filter time constant [s]"; Ts "Sampling time [s]"; x0 "Initial input"; y0 "Initial output"
      mask help: Discrete first order low pass filter derived from a continous filter by bilinear transformation.
  Low pass filter Q : Subsystem  mask(Discrete first order low pass filter){tau=sm.Q_measure, Ts=Ts, x0=0, y0=0}
      mask prompts: tau "Filter time constant [s]"; Ts "Sampling time [s]"; x0 "Initial input"; y0 "Initial output"
      mask help: Discrete first order low pass filter derived from a continous filter by bilinear transformation.
  Measure1 : powerlib/Measurements/Three-Phase V-I Measurement  VoltageMeasurement=phase-to-ground  SetLabelV=off  LabelV=genOut  Vpu=off  VpuLL=off  CurrentMeasurement=yes  SetLabelI=off  LabelI=genCurrentOut  Ipu=off  Pbase=1e3  Vbase=380  OutputType=Magnitude  PhasorSimulation=off  PSBequivalent=0
  Measure3 : powerlib/Measurements/Three-Phase V-I Measurement  VoltageMeasurement=phase-to-ground  SetLabelV=off  LabelV=genOut  Vpu=off  VpuLL=off  CurrentMeasurement=yes  SetLabelI=off  LabelI=genCurrentOut  Ipu=off  Pbase=1e3  Vbase=380  OutputType=Magnitude  PhasorSimulation=off  PSBequivalent=0
  "Power (dq0, Instantaneous)" : powerlib_meascontrol/Measurements/Power (dq0, Instantaneous)
  Product{,1..5} (6 alike) : Product
  Scope : Scope
  Series RLC Branch : powerlib/Elements/Series RLC Branch  LConnTagsString=__new0  RConnTagsString=__new0  BranchType=RL  Resistance=sm.R  Inductance=sm.L  SetiL0=off  InitialCurrent=0  Capacitance=1e-6  Setx0=off  InitialVoltage=0  Measurements=None
  Series RLC Branch1 : powerlib/Elements/Series RLC Branch  LConnTagsString=__new0  RConnTagsString=__new0  BranchType=RL  Resistance=sm.R  Inductance=sm.L  SetiL0=off  InitialCurrent=0  Capacitance=1e-6  Setx0=off  InitialVoltage=0  Measurements=None
  Series RLC Branch2 : powerlib/Elements/Series RLC Branch  LConnTagsString=__new0  RConnTagsString=__new0  BranchType=RL  Resistance=sm.R  Inductance=sm.L  SetiL0=off  InitialCurrent=0  Capacitance=1e-6  Setx0=off  InitialVoltage=0  Measurements=None
  Sqrt1 : Sqrt  SaturateOnIntegerOverflow=on
  Sqrt2 : Sqrt  SaturateOnIntegerOverflow=on
  Sqrt3 : Sqrt  SaturateOnIntegerOverflow=on
  Sum : Sum
  Sum1 : Sum
  Sum2 : Sum
  Terminator : Terminator
  Terminator1 : Terminator
  abc to dq0 : powerlib_meascontrol/Transformations/abc to dq0  Alignment=Aligned with phase A axis
  abc to dq1 : powerlib_meascontrol/Transformations/abc to dq0  Alignment=Aligned with phase A axis
  abc to dq2 : powerlib_meascontrol/Transformations/abc to dq0  Alignment=Aligned with phase A axis
  powerCalcAndFilt1 : Subsystem
  sinusRefGen : Subsystem
  L1 : PMIOPort  Port=1  Side=Right
  L2 : PMIOPort  Port=2  Side=Right
  L3 : PMIOPort  Port=3  Side=Right
  N : PMIOPort  Port=4  Side=Right
  wt1 : Outport
  sm_gen_measure : Outport  Port=2
  wires:
  abc to dq1/1 -> Gain8/1, "Power (dq0, Instantaneous)"/2
  Gain13/1 -> Demux2/1, Demux5/1
  LP filter 3 2/1(out) -> Bus Creator3/3  "0"
  LP filter 6/1(out) -> Bus Creator3/2  "vq"
  LP filter 5/1(out) -> Bus Creator3/1  "vd"
  Bus Creator3/1 -> Bus Creator4/16  "BackEmf_dqo_filt [pu]"
  Demux5/1 -> LP filter 5/1(in)
  Demux5/3 -> LP filter 3 2/1(in)
  Demux5/2 -> LP filter 6/1(in)
  Gain14/1 -> Bus Creator4/14  "BackEmf_filt [rms]"
  [wt] -> abc to dq2/2
  LP filter 4/1(out) -> Bus Creator4/15, Gain14/1  "BackEmf_filt [pu]"
  Sqrt3/1 -> LP filter 4/1(in)  "v_pu"
  Sum2/1 -> Sqrt3/1
  Product5/1 -> Sum2/2
  Demux2/2 -> Product5/1, Product5/2
  Product4/1 -> Sum2/1
  Demux2/1 -> Product4/1, Product4/2
  [Emf_abc] -> abc to dq2/1
  Gain12/1 -> Gain13/1
  abc to dq2/1 -> Gain12/1
  Frequency [pu]/1 -> Gain/1, [sm_freq_pu]
  [sm_backEmfActual_pu] -> Bus Creator4/13  "sm_backEmfActual [pu]"
  [sm_freq_pu] -> Bus Creator4/12  "sm_freq [pu]"
  Gain11/1 -> sinusRefGen/1(GenBackEmf [VrmsLL])
  [sm_backEmfPowerMeasure_pu] -> Bus Creator4/11  "sm_backEmfPowerMeasure_pu"
  Bus Creator4/1 -> sm_gen_measure/1  "sm_genMeas"
  Low pass filter Q/1(out) -> Gain2/1, Bus Creator4/10  "Qgen_VAr"
  Low pass filter P1/1(out) -> Gain7/1, Bus Creator4/8  "Pgen_W"
  "Power (dq0, Instantaneous)"/2 -> Low pass filter Q/1(in)
  "Power (dq0, Instantaneous)"/1 -> Low pass filter P1/1(in)
  Bus Creator/1 -> Scope/1
  Gain5/1 -> Demux/1, Demux1/1, [Vdq0]  "Vgen_dqo_filt [pu]"
  Gain10/1 -> Bus Creator4/4  "Igen_abc [rms]"
  LP filter 3 1/1(out) -> Bus Creator2/3  "I0"
  LP filter 3/1(out) -> Bus Creator2/2  "Iq"
  LP filter 1/1(out) -> Bus Creator2/1  "Id"
  Bus Creator2/1 -> Bus Creator4/6  "Igen_dqo_filt [pu]"
  Demux4/1 -> LP filter 1/1(in)
  Demux4/3 -> LP filter 3 1/1(in)
  Demux4/2 -> LP filter 3/1(in)
  [wt] -> abc to dq1/2
  LP filter 67/1(out) -> Bus Creator4/5, Gain10/1  "Igen_filt [pu]"
  Sqrt2/1 -> LP filter 67/1(in)  "v_pu"
  Sum1/1 -> Sqrt2/1
  Product3/1 -> Sum1/2
  Demux3/2 -> Product3/1, Product3/2
  Product2/1 -> Sum1/1
  Demux3/1 -> Product2/1, Product2/2
  Gain9/1 -> Demux3/1, Demux4/1, [Idq0]
  [Iabc] -> abc to dq1/1
  Gain8/1 -> Gain9/1
  Measure1/2 -> [Iabc], Bus Creator/2
  Gain6/1 -> Bus Creator4/1  "Vgen_filt [rms]"
  Measure1/1 -> [Vabc], Bus Creator/1
  "LP filter 3 "/1(out) -> Bus Creator1/3  "0"
  LP filter 2/1(out) -> Bus Creator1/2  "vq"
  "LP filter "/1(out) -> Bus Creator1/1  "vd"
  Bus Creator1/1 -> Bus Creator4/3  "Vgen_dqo_filt [pu]"
  Demux1/1 -> "LP filter "/1(in)
  Demux1/3 -> "LP filter 3 "/1(in)
  Demux1/2 -> LP filter 2/1(in)
  [wt] -> abc to dq0/2
  powerCalcAndFilt1/2(Q_filt1) -> Terminator/1
  Gain1/1 -> [sm_backEmfPowerMeasure_pu]
  powerCalcAndFilt1/1(P_filt) -> Gain1/1
  Measure3/2 -> powerCalcAndFilt1/2(Iabc)
  Measure3/1 -> powerCalcAndFilt1/1(Vabc), [Emf_abc]
  LP filter 66/1(out) -> Bus Creator4/2, Gain6/1  "Vgen_filt [pu]"
  Sqrt1/1 -> LP filter 66/1(in)  "v_pu"
  Sum/1 -> Sqrt1/1
  Product1/1 -> Sum/2
  Demux/2 -> Product1/1, Product1/2
  Product/1 -> Sum/1
  Demux/1 -> Product/1, Product/2
  [Vabc] -> abc to dq0/1
  Gain4/1 -> Gain5/1
  Gain3/1 -> Discrete-Time Integrator1/1
  Gain/1 -> [sm_freq_Hz], sinusRefGen/2(freq Hz), Gain3/1  "f"
  abc to dq0/1 -> Gain4/1, "Power (dq0, Instantaneous)"/1
  Discrete-Time Integrator1/1 -> wt1/1, [wt]
  Gain2/1 -> Bus Creator4/9  "Qgen_pu"
  Gain7/1 -> Bus Creator4/7  "Pgen_pu"
  sinusRefGen/3(c) -> B1/1
  sinusRefGen/2(b) -> B/1
  sinusRefGen/1(a) -> A/1
  Phase [rad]/1 -> sinusRefGen/3(phase (rad))
  GenBackEmf [pu]/1 -> Gain11/1, [sm_backEmfActual_pu]
  phaseSkiftIndividual/1 -> sinusRefGen/5(phaseSkiftIndividual)
  deltaAmplitudeIndividual/1 -> sinusRefGen/4(deltaAmplitudeIndividual)
  Demux2/3 -> Terminator1/1
  connections:
  Series RLC Branch/LConn1 -- Measure3/RConn1
  Series RLC Branch1/LConn1 -- Measure3/RConn2
  Series RLC Branch2/LConn1 -- Measure3/RConn3
  L1/RConn1 -- Measure1/RConn1
  L2/RConn1 -- Measure1/RConn2
  L3/RConn1 -- Measure1/RConn3
  Series RLC Branch2/RConn1 -- Measure1/LConn3
  Series RLC Branch1/RConn1 -- Measure1/LConn2
  Series RLC Branch/RConn1 -- Measure1/LConn1
  Measure3/LConn3 -- B1/RConn1
  Measure3/LConn2 -- B/RConn1
  A/RConn1 -- Measure3/LConn1
  B/LConn1 -- B1/LConn1 -- N/RConn1 -- A/LConn1

== system Just_The_Electrical_model/Electric system/Turbine Governor1 ==
  FCRN_Case2 : Inport
  FCRN_Case3 : Inport  Port=2
  EnableActuatorDelay : Inport  Port=3
  Speed_ref (pu) : Inport  Port=4
  deltaSpeedRef (pu) : Inport  Port=5
  Speed_feedback (pu) : Inport  Port=6
  pRef (pu) : Inport  Port=7
  Constant10 : Constant  Value=governor.FCR.N.MaxDroopContrib_case3  SampleTime=-1
  Constant11 : Constant  Value=governor.FCR.N.MinDroopContrib_case3  SampleTime=-1
  Constant12 : Constant  Value=governor.FCR.N.MinDroopContrib_case1  SampleTime=-1
  Constant13 : Constant  Value=governor.FCR.N.MinDroopContrib_case2  SampleTime=-1
  Constant2 : Constant  Value=governor.FCR.D.kp  SampleTime=governor.FCR.Ts
  Constant25 : Constant  Value=governor.FCR.N.kp_case1  SampleTime=-1
  Constant26 : Constant  Value=governor.FCR.N.kp_case2  SampleTime=-1
  Constant27 : Constant  Value=governor.FCR.N.kp_case3  SampleTime=-1
  Constant3 : Constant  Value=governor.FCR.D.MaxDroopContrib  SampleTime=governor.FCR.Ts
  Constant4 : Constant  Value=governor.FCR.D.MinDroopContrib  SampleTime=governor.FCR.Ts
  Constant7 : Constant  Value=0
  Constant8 : Constant  Value=governor.FCR.N.MaxDroopContrib_case1  SampleTime=-1
  Constant9 : Constant  Value=governor.FCR.N.MaxDroopContrib_case2  SampleTime=-1
  Droop1 : Sum
  Droop_controller FCRN : pwrsysBasic/Droop_controller   Ts=governor.FCR.Ts  Outmax=1  Outmin=-1  Refmax=1  Refmin=0  Kd=0  Tr=1  flp=governor.flp  DB=governor.FCR.N.DB  flp_comp=governor.flp  Compmax=1.2  Compini=1  Compmin=0.8
  Droop_controller_FCRD : pwrsysBasic/Droop_controller   Ts=governor.FCR.Ts  Outmax=governor.FCR.D.MaxOutput  Outmin=governor.FCR.D.MinOutput  Refmax=governor.FCR.D.MaxOutput  Refmin=governor.FCR.D.MinOutput  Kd=0  Tr=1  flp=governor.flp  DB=governor.FCR.D.DB  flp_comp=governor.flp  Compmax=1.2  Compini=1  Compmin=0.8
  LP filter power : Subsystem  mask(Discrete first order low pass filter){tau=governor.LPfilterActuator.T1, Ts=Ts, x0=0, y0=0}
      mask prompts: tau "Filter time constant [s]"; Ts "Sampling time [s]"; x0 "Initial input"; y0 "Initial output"
      mask help: Discrete first order low pass filter derived from a continous filter by bilinear transformation.
  LP filter power2 : Subsystem  mask(Discrete first order low pass filter){tau=governor.LPfilterActuator.T2, Ts=Ts, x0=0, y0=0}
      mask prompts: tau "Filter time constant [s]"; Ts "Sampling time [s]"; x0 "Initial input"; y0 "Initial output"
      mask help: Discrete first order low pass filter derived from a continous filter by bilinear transformation.
  Saturation1 : Saturate  UpperLimit=1  LowerLimit=0
  Speed_err1 : Sum  Inputs=-+
  Sum : Sum  Inputs=|++
  Switch1 : Switch  Criteria=u2 > Threshold
  Switch{2..7} (6 alike) : Switch  Threshold=0.5
  output (pu) : Outport
  wires:
  EnableActuatorDelay/1 -> Switch1/2
  Speed_err1/1 -> Droop_controller FCRN/1, Droop_controller_FCRD/1
  Droop1/1 -> Speed_err1/1
  Speed_ref (pu)/1 -> Droop1/1
  Sum/1 -> Saturation1/1
  Switch1/1 -> output (pu)/1
  Speed_feedback (pu)/1 -> Droop_controller_FCRD/6, Droop_controller FCRN/6, Speed_err1/2
  deltaSpeedRef (pu)/1 -> Droop1/2
  pRef (pu)/1 -> Droop_controller_FCRD/5
  Constant2/1 -> Droop_controller_FCRD/2
  Constant3/1 -> Droop_controller_FCRD/3
  Constant4/1 -> Droop_controller_FCRD/4
  Droop_controller_FCRD/1 -> Sum/2
  Droop_controller FCRN/1 -> Sum/1
  [FCRNKp] -> Droop_controller FCRN/2
  [FCRNmax] -> Droop_controller FCRN/3
  [FCRNmin] -> Droop_controller FCRN/4
  Constant7/1 -> Droop_controller FCRN/5
  Saturation1/1 -> LP filter power/1(in), Switch1/3
  [FCRNCase2] -> Switch2/2
  Constant25/1 -> Switch2/3
  Constant26/1 -> Switch2/1
  Switch2/1 -> Switch3/3
  [FCRNCase3] -> Switch3/2
  Constant27/1 -> Switch3/1
  Switch3/1 -> [FCRNKp]
  FCRN_Case2/1 -> [FCRNCase2]
  FCRN_Case3/1 -> [FCRNCase3]
  [FCRNCase2] -> Switch4/2
  Constant8/1 -> Switch4/3
  Constant9/1 -> Switch4/1
  Switch4/1 -> Switch5/3
  [FCRNCase3] -> Switch5/2
  Constant10/1 -> Switch5/1
  Switch5/1 -> [FCRNmax]
  [FCRNCase2] -> Switch6/2
  Constant12/1 -> Switch6/3
  Constant13/1 -> Switch6/1
  Switch6/1 -> Switch7/3
  [FCRNCase3] -> Switch7/2
  Constant11/1 -> Switch7/1
  Switch7/1 -> [FCRNmin]
  LP filter power/1(out) -> LP filter power2/1(in)
  LP filter power2/1(out) -> Switch1/1
